simulink model "ball_on_beam_nonlinear_model_reference"  (R2021a)
settings: Solver=VariableStepAuto  StartTime=0.0  StopTime=1.4  RelTol=1e-3
settings Model: Creator=muellerb  LastModifiedBy=muellerb

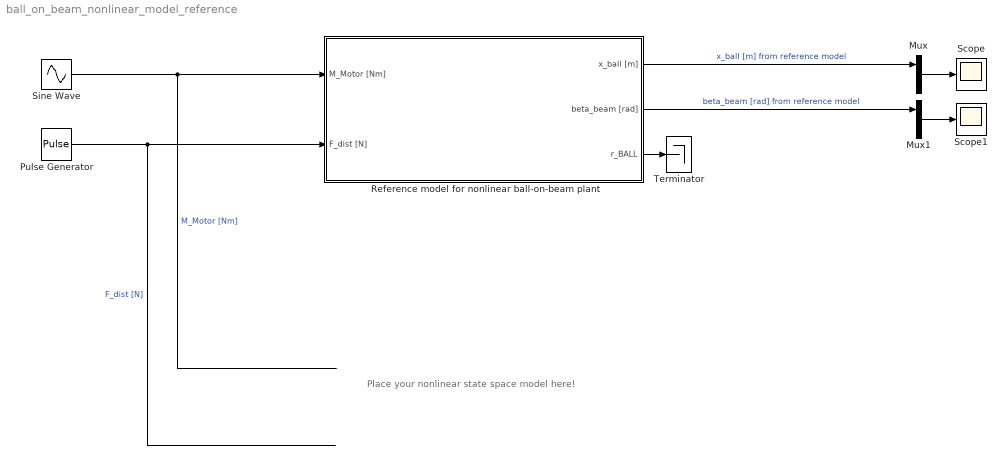
== system ball_on_beam_nonlinear_model_reference ==
  note: Place your nonlinear state space model here!
  Mux : Mux  Inputs=2
  Mux1 : Mux  Inputs=2
  Pulse Generator : DiscretePulseGenerator  PulseType=Time based  Amplitude=0.15  Period=0.5  PulseWidth=50  PhaseDelay=0.25
  Reference model for nonlinear ball-on-beam plant : Subsystem  mask(Nonlinear BALL_ON_BEAM model){r_BALL=0.0125, J_BALL=4.00e-06, m_BALL=0.064, G=9.81, J_BEAM=2.9e-3}
      mask prompts: r_BALL "Radius of the ball r_ball [m]"; J_BALL "Moment of inertia of the ball J_ball [kgm^2] (with respect to axis of symmetry)"; m_BALL "Mass of ball m_ball [kg]"; G "Gravity acceleration g [m/s^2]"; J_BEAM "Moment of inertia of the beam J_beam [kgm^2] (with respect to the axis of rotation)"
      mask help: Nonlinear model of ball-on-beam setup (without restrictions on input or state variables)
      mask Display: image('$imagefile'); % Use "Edit Image" on toolstrip to change.
  Scope : Scope
  Scope1 : Scope
  Sine Wave : Sin  Amplitude=0.01  Frequency=2*pi  Phase=pi/2  SampleTime=0
  Terminator : Terminator
  wires:
  Sine Wave/1 -> Reference model for nonlinear ball-on-beam plant/1(M_Motor [Nm])  "M_Motor [Nm]"
  Pulse Generator/1 -> Reference model for nonlinear ball-on-beam plant/2(F_dist [N])  "F_dist [N]"
  Mux/1 -> Scope/1
  Mux1/1 -> Scope1/1
  Reference model for nonlinear ball-on-beam plant/3(r_BALL) -> Terminator/1
  Reference model for nonlinear ball-on-beam plant/1(x_ball [m]) -> Mux/1  "x_ball [m] from reference model"
  Reference model for nonlinear ball-on-beam plant/2(beta_beam [rad]) -> Mux1/1  "beta_beam [rad] from reference model"
  ? -> Mux/2  "x_ball [m] from your model"
  ? -> Mux1/2  "beta_beam [rad] from your model"

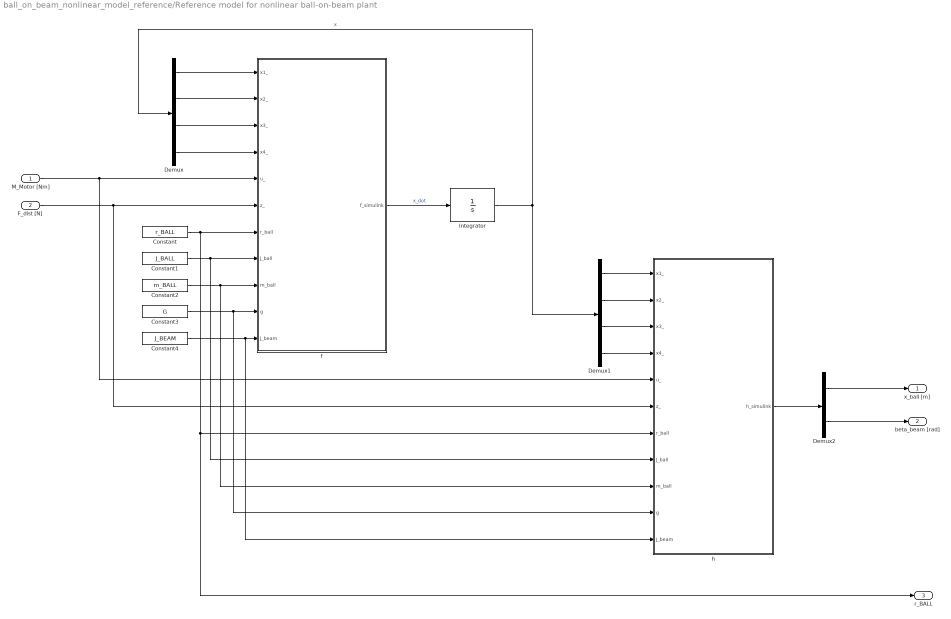
== system ball_on_beam_nonlinear_model_reference/Reference model for nonlinear ball-on-beam plant ==
  M_Motor [Nm] : Inport
  F_dist [N] : Inport  Port=2
  Constant : Constant  Value=r_BALL
  Constant1 : Constant  Value=J_BALL
  Constant2 : Constant  Value=m_BALL
  Constant3 : Constant  Value=G
  Constant4 : Constant  Value=J_BEAM
  Demux : Demux
  Demux1 : Demux
  Demux2 : Demux  Outputs=2
  Integrator : Integrator
  f : MATLAB Function  TreatAsAtomicUnit=on
  h : MATLAB Function  TreatAsAtomicUnit=on
  x_ball [m] : Outport
  beta_beam [rad] : Outport  Port=2
  r_BALL : Outport  Port=3
  wires:
  Demux2/1 -> x_ball [m]/1
  M_Motor [Nm]/1 -> h/5(u_), f/5(u_)
  f/1(f_simulink) -> Integrator/1  "x_dot"
  h/1(h_simulink) -> Demux2/1
  Demux/3 -> f/3(x3_)
  Constant1/1 -> h/8(J_ball), f/8(J_ball)
  Demux/1 -> f/1(x1_)
  Integrator/1 -> Demux/1, Demux1/1  "x"
  F_dist [N]/1 -> h/6(z_), f/6(z_)
  Demux1/1 -> h/1(x1_)
  Constant4/1 -> h/11(J_beam), f/11(J_beam)
  Constant3/1 -> h/10(g), f/10(g)
  Constant/1 -> r_BALL/1, h/7(r_ball), f/7(r_ball)
  Demux2/2 -> beta_beam [rad]/1
  Constant2/1 -> h/9(m_ball), f/9(m_ball)
  Demux/2 -> f/2(x2_)
  Demux/4 -> f/4(x4_)
  Demux1/2 -> h/2(x2_)
  Demux1/3 -> h/3(x3_)
  Demux1/4 -> h/4(x4_)

== matlab function ball_on_beam_nonlinear_model_reference/Reference model for nonlinear ball-on-beam plant/h ==
  data: x1_ input; h_simulink output; x2_ input; x3_ input; x4_ input; u_ input; z_ input; r_ball input; J_ball input; m_ball input; g input; J_beam input
function h_simulink = h(x1_,x2_,x3_,x4_,u_,z_,r_ball,J_ball,m_ball,g,J_beam)
%#codegen

%    This function was generated by the Symbolic Math Toolbox version 8.7.
%    28-Nov-2023 16:51:32

h_simulink = [x1_;...
    x3_];

== matlab function ball_on_beam_nonlinear_model_reference/Reference model for nonlinear ball-on-beam plant/f ==
  data: x1_ input; f_simulink output; x2_ input; x3_ input; x4_ input; u_ input; z_ input; r_ball input; J_ball input; m_ball input; g input; J_beam input
function f_simulink = f(x1_,x2_,x3_,x4_,u_,z_,r_ball,J_ball,m_ball,g,J_beam)
%#codegen

%    This function was generated by the Symbolic Math Toolbox version 8.7.
%    28-Nov-2023 16:51:32

t2 = cos(x3_);
t3 = sin(x3_);
t4 = m_ball.^2;
t5 = r_ball.^2;
t6 = x1_.^2;
t7 = x4_.^2;
t8 = m_ball.*t6;
t9 = J_beam+t8;
t10 = 1.0./t9;
f_simulink = [x2_;...
    (r_ball.*t10.*(J_ball.*u_+J_beam.*r_ball.*z_+m_ball.*t5.*u_+r_ball.*t8.*z_+r_ball.*t4.*t7.*x1_.^3+r_ball.^3.*t4.*t7.*x1_-J_beam.*g.*m_ball.*r_ball.*t3-J_ball.*g.*m_ball.*t2.*x1_+J_beam.*m_ball.*r_ball.*t7.*x1_+J_ball.*m_ball.*r_ball.*t7.*x1_-J_ball.*m_ball.*x1_.*x2_.*x4_.*2.0-g.*r_ball.*t3.*t4.*t6-g.*t2.*t4.*t5.*x1_-t4.*t5.*x1_.*x2_.*x4_.*2.0))./(J_ball+m_ball.*t5);x4_;t10.*(u_-g.*m_ball.*t2.*x1_+m_ball.*r_ball.*t7.*x1_-m_ball.*x1_.*x2_.*x4_.*2.0)];
